simulink model "VFlexP_small"  (R2026a)
settings: Solver=ode23tb  StopTime=2  FixedStep=5e-5
model workspace (MAT data in the model file):
  DCop_DCBUCK : object (value not decoded)
  Grid_CCVSC_idx = [2; 3; 4; 5; 6; 7; 8; 9; 10; 11; 12]
  Grid_CCVSCs = 1
  Grid_CCVSCs_buses = 1
  Grid_CCVSCs_toM = [0 1 0 0 0 0 0 0 0 0 0 0 ... (781 elements, 71x11)]
  Grid_C_Lines = 0
  Grid_Cbuses = [0.00666666666667 0.00666666666667]
  Grid_DC : object (value not decoded)
  Grid_DCop_DCBUCK : object (value not decoded)
  Grid_DCop_DC_PES : object (value not decoded)
  Grid_DFIGs = 1
  Grid_DFIGs_buses = 1
  Grid_DGs : string (value not decoded)
  Grid_From_buses = 1
  Grid_GFls = 1
  Grid_GFls_buses = 1
  Grid_GFr_idx = 1
  Grid_GFrs = 1
  Grid_GFrs_buses = 1
  Grid_GFrs_toM = [1; 0]
  Grid_IG_idx = 1
  Grid_IGs = 1
  Grid_IGs_buses = 1
  Grid_IGs_toM = [1; 0; 0]
  Grid_L_Lines = 0.05
  Grid_L_Loads = [0 0]
  Grid_Lines_fromM : object (value not decoded)
  Grid_Lines_toM : object (value not decoded)
  Grid_Load_buses = [1; 2]
  Grid_Load_busesDC = []
  Grid_MSGs = 1
  Grid_MSGs_buses = 1
  Grid_Nbuses = 2
  Grid_PQ_gen = 3
  Grid_Ploads = [0.0075 0.0075]
  Grid_PloadsDC = []
  Grid_Ps_lf = 0.51232912
  Grid_Qloads = [0 0]
  Grid_Qs_lf = -0.00723209333333
  Grid_R_Lines = 0.005
  Grid_R_Loads = [2 2]
  Grid_R_Loads_DC = 0
  Grid_Rcf = [150 150]
  Grid_SCs = 1
  Grid_SCs_buses = 1
  Grid_SG_idx = 1
  Grid_SGs = 1
  Grid_SGs_buses = 1
  Grid_SGs_toM = [1; 0]
  Grid_To_buses = 2
  Grid_VCVSC_idx = [1; 2; 3; 4; 5; 6; 7; 8; 9; 10; 11; 12]
  Grid_VCVSCs = 1
  Grid_VCVSCs_buses = [1; 2; 3; 6; 8; 9; 12; 58; 59; 60; 63; 65]
  Grid_VCVSCs_toM = [1 0 0 0 0 0 0 0 0 0 0 0 ... (852 elements, 71x12)]
  Grid_VSM_idx = 2
  Grid_VSMs = 1
  Grid_VSMs_buses = 1
  Grid_VSMs_toM = [0; 1]
  Grid_admitt_matrix = [2.15353135314-19.7953135314i  -1.9801980198+19.801980198i; -1.9801980198+19.801980198i  2.15353135314-19.7953135314i]
  Grid_admitt_matrix_noloads = [1.98686468647-19.7953135314i  -1.9801980198+19.801980198i; -1.9801980198+19.801980198i  1.98686468647-19.7953135314i]
  Grid_bus = [1; 2]
  Grid_busDC_complexity = 1
  Grid_busDC_complexity_PF = 2
  Grid_bus_complexity = [1 1]
  Grid_bus_complexity_PF = [1 1]
  Grid_buses_lf = 1
  Grid_conductance_matrix = 0.00666666666667
  Grid_conductance_matrix_noloads = 0.00666666666667
  Grid_fref : object (value not decoded)
  Grid_gen_static_params : mBase (value not decoded)
  Grid_iPs_lf = 1.95187031336
  Grid_iQs_lf = -138.272551792
  Grid_iadmitt_matrix = [2.88165849328-0.0982918688642i  2.87905051706-0.123273862303i; 2.87905051706-0.123273862303i  2.88165849328-0.0982918688642i]
  Grid_iadmitt_matrix_noloads = [37.5012524798-37.4874983544i  37.4987475202-37.5125016456i; 37.4987475202-37.5125016456i  37.5012524798-37.4874983544i]
  Grid_iconductance_matrix = 150
  Grid_iconductance_matrix_noloads = 150
  Grid_init_OK_bool = 1
  Grid_intconv_PF : object (value not decoded)
  Grid_lf_op : op_report (value not decoded)
  Grid_lineDC_complexity = []
  Grid_lineDC_complexity_PF = []
  Grid_line_complexity = 1
  Grid_line_complexity_PF = 3
  Grid_loadDC_complexity = []
  Grid_loadDC_complexity_PF = []
  Grid_load_complexity = [3 3]
  Grid_load_complexity_PF = [4 4]
  Grid_opDC_CCVSC : object (value not decoded)
  Grid_opDC_VSM : object (value not decoded)
  Grid_opGFr : object (value not decoded)
  Grid_opVCVSC : object (value not decoded)
  Grid_op_CCVSC : object (value not decoded)
  Grid_op_IG : object (value not decoded)
  Grid_op_SG : object (value not decoded)
  Grid_op_VSM : object (value not decoded)
  Grid_shift_lines = 0
  Grid_tap_lines = 1
  Grid_v_buses_mod = [1 1]
  LinsysParamChangeStruct : Param1 (value not decoded)
  Lline = 0.01
  Rline = 1e-05
  linsys : object (value not decoded)
values from neighbouring files (symbols this model uses):
  block_idx = evalin(mdlWks, [bvarname Generators{i} '_idx'])    [fun_init_units_callback.m]
  Fb = areas    [fun_MATPOWER_to_Excel.m]
  Fi = evalin('base', get_param(block, 'Fi'))    [fun_init_GFr.m]    (also in fun_init_intconv_DC_VSM.m)
  Lf = evalin('base', get_param(block, 'Lf'))    [fun_init_GFr.m]    (also in fun_init_intconv_DC_VSM.m)
  Rf = evalin('base', get_param(block, 'Rf'))    [fun_init_GFr.m]    (also in fun_init_intconv_DC_VSM.m)
symbols that are objects in the model workspace (value not decoded): Grid_DCop_DC_PES, Grid_DCop_DCBUCK, Grid_op_CCVSC, Grid_op_IG, Grid_op_SG, Grid_op_VSM, Grid_opDC_CCVSC, Grid_opDC_VSM, Grid_opGFr, Grid_opVCVSC
undefined symbols (not defined in the file or in its folder): block_buses_DC, CCVSC_idx, Cf, costs, costs2, DFIGs_nodes, DiscIntNeverNeededParam, entity, From_nodes, grid_linsys, Grid_op_DFIG, Grid_op_DFIG_PQ, Grid_op_MSG, Grid_op_SC, Grid_op_VCVSC, Hv, initial_states_grid, Kic, Kiv, Kp_theta, Kp_w, Kpc, Kpv, last_send, Lc, m, Matrix_flux_to_i, mD, mp, MSGs_buses, Nbuses_DC, nq, op_VCVSC, Psche, Rc, rkq1, rkq2, SCs_buses, SCs_nodes, sec_control_structure, set_asked, set_DG_up, set_extra_satur, set_sending_cost, SGs_buses, SGs_nodes, Tf, To_nodes, VI_L, VI_R, WOF_Tf, xkq1, xkq2
libraries: simulink x1045, eeGeneralControl x12, eeTransforms x1, sl_discontinuities x1
(part 25 of 50)

== system VFlexP_small/Grid/Loadflow/Loads/dynamic/to_all_Loads1 ==
  In1 : Inport
  Assignment : Assignment  DiagnosticForDimensions=Warning  IndexOptions=Index vector (dialog)  Indices=find(load_complexity_PF == 1)  OutputSizes=1
  Zero : Constant  Value=zeros(1,length(L_Loads))  VectorParams1D=off  OutDataTypeStr=Inherit: Inherit via back propagation
  id : Outport
  wires:
  Assignment/1 -> id/1
  In1/1 -> Assignment/2
  Zero/1 -> Assignment/1

== system VFlexP_small/Grid/Loadflow/Loads/dynamic PQ/to_all_Loads ==
  In1 : Inport
  Assignment : Assignment  DiagnosticForDimensions=Warning  IndexOptions=Index vector (dialog)  Indices=find(load_complexity_PF == 5)  OutputSizes=1
  Zero : Constant  Value=zeros(1,length(L_Loads))  VectorParams1D=off  OutDataTypeStr=Inherit: Inherit via back propagation
  Out1 : Outport
  wires:
  Zero/1 -> Assignment/1
  In1/1 -> Assignment/2
  Assignment/1 -> Out1/1

== system VFlexP_small/Grid/Loadflow/Loads/dynamic PQ/to_all_Loads1 ==
  In1 : Inport
  Assignment : Assignment  DiagnosticForDimensions=Warning  IndexOptions=Index vector (dialog)  Indices=find(load_complexity_PF == 5)  OutputSizes=1
  Zero : Constant  Value=zeros(1,length(L_Loads))  VectorParams1D=off  OutDataTypeStr=Inherit: Inherit via back propagation
  Out1 : Outport
  wires:
  Assignment/1 -> Out1/1
  In1/1 -> Assignment/2
  Zero/1 -> Assignment/1

== system VFlexP_small/Grid/Loadflow/Loads/static/to_all_Loads ==
  In1 : Inport
  Assignment : Assignment  DiagnosticForDimensions=Warning  IndexOptions=Index vector (dialog)  Indices=find(load_complexity_PF == 2)  OutputSizes=1
  Zero : Constant  Value=zeros(1,length(L_Loads))  VectorParams1D=off  OutDataTypeStr=Inherit: Inherit via back propagation
  id : Outport
  wires:
  Zero/1 -> Assignment/1
  In1/1 -> Assignment/2
  Assignment/1 -> id/1

== system VFlexP_small/Grid/Loadflow/Loads/static/to_all_Loads1 ==
  In1 : Inport
  Assignment : Assignment  DiagnosticForDimensions=Warning  IndexOptions=Index vector (dialog)  Indices=find(load_complexity_PF == 2)  OutputSizes=1
  Zero : Constant  Value=zeros(1,length(L_Loads))  VectorParams1D=off  OutDataTypeStr=Inherit: Inherit via back propagation
  id : Outport
  wires:
  Assignment/1 -> id/1
  In1/1 -> Assignment/2
  Zero/1 -> Assignment/1

== system VFlexP_small/Grid/Loadflow/Loads/static omega/to_all_Loads ==
  In1 : Inport
  Assignment : Assignment  DiagnosticForDimensions=Warning  IndexOptions=Index vector (dialog)  Indices=find(load_complexity_PF == 3)  OutputSizes=1
  Zero : Constant  Value=zeros(1,length(L_Loads))  VectorParams1D=off  OutDataTypeStr=Inherit: Inherit via back propagation
  id : Outport
  wires:
  Zero/1 -> Assignment/1
  In1/1 -> Assignment/2
  Assignment/1 -> id/1

== system VFlexP_small/Grid/Loadflow/Loads/static omega/to_all_Loads1 ==
  In1 : Inport
  Assignment : Assignment  DiagnosticForDimensions=Warning  IndexOptions=Index vector (dialog)  Indices=find(load_complexity_PF == 3)  OutputSizes=1
  Zero : Constant  Value=zeros(1,length(L_Loads))  VectorParams1D=off  OutDataTypeStr=Inherit: Inherit via back propagation
  id : Outport
  wires:
  Assignment/1 -> id/1
  In1/1 -> Assignment/2
  Zero/1 -> Assignment/1

== system VFlexP_small/Grid/Dynamic/DCAC converters/DC_CCVSC/CC/dynamic ==
  idref : Inport
  iqref : Inport  Port=2
  vod : Inport  Port=3
  voq : Inport  Port=4
  omega : Inport  Port=5
  "Lf " : Gain  Gain=dparams.Lf
  Lf1 : Gain  Gain=dparams.Lf
  PId : Subsystem
  PIq : Subsystem
  Product : Product
  Product3 : Product
  RL : Subsystem  Variant=on  VariantControlMode=label  LabelModeActiveChoice=dynamic  mask(Line){dynamic=Dynamic, R=dparams.Rf, L=dparams.Lf, fbase=fb}
      mask prompts: dynamic "Dynamic behavior"; R "Series resistance (p.u.)"; L "Inductance (p.u.)"; fbase "Base frequency (Hz)"
      mask init: same as VFlexP_small/Grid/Loadflow/Generators/RL out
      mask Help: web('Documentation/RL.html')
      mask TypeOptions dynamic: Static | Dynamic | Static omega
  Sum1 : Sum  Inputs=++|
  Sum2 : Sum  Inputs=++|
  Sum8 : Sum  Inputs=-+|
  Sum9 : Sum  Inputs=|++
  idiref : Outport
  iqiref : Outport  Port=2
  vid : Outport  Port=3
  viq : Outport  Port=4
  wires:
  PId/1(Out1) -> Sum8/2
  idref/1 -> PId/1(ref)  "idref"
  RL/1(id) -> idiref/1, Lf1/1, PId/2(y)
  Sum2/1 -> viq/1, RL/3(v_in_q)
  Sum1/1 -> vid/1, RL/1(v_in_d)
  [voq] -> RL/4(v_out_q)
  [vod] -> RL/2(v_out_d)
  vod/1 -> [vod]  "iod"
  voq/1 -> [voq]  "ioq"
  omega/1 -> [omega]  "omega"
  [voq] -> Sum2/1
  [vod] -> Sum1/1
  Sum9/1 -> Sum2/2
  Sum8/1 -> Sum1/2
  iqref/1 -> PIq/1(ref)  "iqref"
  Product/1 -> Sum8/1
  [omega] -> Product/2
  Lf1/1 -> Product3/2
  Product3/1 -> Sum9/2
  "Lf "/1 -> Product/1
  [omega] -> Product3/1  "omega"
  PIq/1(Out1) -> Sum9/1
  RL/2(iq) -> "Lf "/1, PIq/2(y), iqiref/1
  [omega] -> RL/5(omega)  "omega"

== system VFlexP_small/Grid/Dynamic/DCAC converters/DC_CCVSC/CC/static ==
  idref : Inport
  iqref : Inport  Port=2
  vod : Inport  Port=3
  voq : Inport  Port=4
  omega : Inport  Port=5
  Terminator2 : Terminator
  idiref : Outport
  iqiref : Outport  Port=2
  vid : Outport  Port=3
  viq : Outport  Port=4
  wires:
  omega/1 -> Terminator2/1  "omega"
  iqref/1 -> iqiref/1  "iqref"
  idref/1 -> idiref/1  "idref"
  vod/1 -> vid/1  "vod"
  voq/1 -> viq/1  "voq"

== system VFlexP_small/Grid/Dynamic/DCAC converters/DC_CCVSC/PC/LPF_d ==
  In1 : Inport
  Gain : Gain  Gain=iTf
  I : Integrator  InitialCondition=v_buses_mod(block_buses)
  Sum4 : Sum  Inputs=|+-
  Out1 : Outport
  wires:
  I/1 -> Out1/1, Sum4/2
  In1/1 -> Sum4/1
  Sum4/1 -> Gain/1
  Gain/1 -> I/1

== system VFlexP_small/Grid/Dynamic/DCAC converters/DC_CCVSC/PC/LPF_q ==
  In1 : Inport
  Gain : Gain  Gain=iTf
  I : Integrator
  Sum4 : Sum  Inputs=|+-
  Out1 : Outport
  wires:
  Sum4/1 -> Gain/1
  In1/1 -> Sum4/1
  I/1 -> Out1/1, Sum4/2
  Gain/1 -> I/1

== system VFlexP_small/Grid/Dynamic/DCAC converters/DC_CCVSC/PC/Saturation ==
  ildref : Inport
  ilqref : Inport  Port=2
  Abs : Abs  ZeroCross=off  SaturateOnIntegerOverflow=off
  Abs1 : Abs  ZeroCross=off  SaturateOnIntegerOverflow=off
  Abs2 : Abs  ZeroCross=off  SaturateOnIntegerOverflow=off
  Divide2 : Product  Inputs=*/
  Divide3 : Product  Inputs=*/
  Gain : Gain  Gain=-1
  Gain3 : Gain  Gain=-1
  Real-Imag to Complex : RealImagToComplex
  Saturation Dynamic : simulink/Discontinuities/Saturation Dynamic  OutMin=[]  OutMax=[]  OutDataTypeStr=Inherit: Same as second input  OutDataType=fixdt(1, 16)  OutScaling=2^-10  DoSatur=off
  Saturation Dynamic1 : simulink/Discontinuities/Saturation Dynamic  OutMin=[]  OutMax=[]  OutDataTypeStr=Inherit: Same as second input  OutDataType=fixdt(1, 16)  OutScaling=2^-10  DoSatur=off
  y : Outport
  y1 : Outport  Port=2
  wires:
  Saturation Dynamic1/1 -> y1/1
  ildref/1 -> Real-Imag to Complex/1, Saturation Dynamic/2, Abs2/1
  Abs2/1 -> Divide2/1
  ilqref/1 -> Real-Imag to Complex/2, Saturation Dynamic1/2, Abs1/1
  Real-Imag to Complex/1 -> Abs/1
  Abs1/1 -> Divide3/1
  Gain3/1 -> Saturation Dynamic/3
  Abs/1 -> Divide2/2, Divide3/2
  Saturation Dynamic/1 -> y/1
  Divide2/1 -> Saturation Dynamic/1, Gain3/1
  Divide3/1 -> Saturation Dynamic1/1, Gain/1
  Gain/1 -> Saturation Dynamic1/3

== system VFlexP_small/Grid/Dynamic/DCAC converters/DC_CCVSC/PLL/dynamic ==
  vq : Inport
  omega : Inport  Port=2
  voutangle : Inport  Port=3
  PLL : Subsystem
  Product : Product
  Selector8 : Selector  InputPortWidth=length(fref.ref_units)  IndexOptions=Index vector (dialog)  Indices=block_fref  OutputSizes=1
  Sum2 : Sum  Inputs=|-+
  Sum3 : Sum  Inputs=+-|
  Terminator : Terminator
  Zero : Constant  Value=0  OutDataTypeStr=Inherit: Inherit via back propagation
  frame : Integrator  InitialCondition=Grid_opDC_CCVSC.frame  UpperSaturationLimit=pi  LowerSaturationLimit=-pi
  theta : Outport
  omega_point : Outport  Port=2
  wires:
  Sum2/1 -> PLL/1(In1)
  Sum3/1 -> Product/1
  PLL/1(Input2) -> Sum3/1, omega_point/1  "omega2"
  Product/1 -> frame/1
  frame/1 -> theta/1  "theta"
  Zero/1 -> Sum2/1
  omega/1 -> Sum3/2  "omega"
  vq/1 -> Sum2/2  "vq"
  voutangle/1 -> Terminator/1
  [omega_base] -> Selector8/1
  Selector8/1 -> Product/2

== system VFlexP_small/Grid/Dynamic/DCAC converters/DC_CCVSC/PLL/static ==
  vq : Inport
  omega : Inport  Port=2
  voutangle : Inport  Port=3
  Gain : Gain  Gain=-1
  Terminator : Terminator
  Terminator1 : Terminator
  Transport Delay : TransportDelay  DelayTime=1e-6  TransDelayFeedthrough=on
  theta : Outport
  omega_point : Outport  Port=2
  wires:
  voutangle/1 -> Gain/1
  omega/1 -> Terminator1/1, omega_point/1  "vq"
  vq/1 -> Terminator/1  "vq"
  Gain/1 -> Transport Delay/1
  Transport Delay/1 -> theta/1

== system VFlexP_small/Grid/Dynamic/DCAC converters/DC_VCVSC/PC/LPF_P ==
  P : Inport
  Gain : Gain  Gain=iTf
  I : Integrator  InitialCondition=Grid_op_VCVSC.States(5,:)
  Sum4 : Sum  Inputs=|+-
  P_f : Outport
  wires:
  I/1 -> Sum4/2, P_f/1
  P/1 -> Sum4/1
  Sum4/1 -> Gain/1
  Gain/1 -> I/1

== system VFlexP_small/Grid/Dynamic/DCAC converters/DC_VCVSC/PC/LPF_Q ==
  Q : Inport
  Gain : Gain  Gain=iTf
  I : Integrator  InitialCondition=Grid_op_VCVSC.States(6,:)
  Sum4 : Sum  Inputs=|+-
  Q_f : Outport
  wires:
  Sum4/1 -> Gain/1
  I/1 -> Sum4/2, Q_f/1
  Q/1 -> Sum4/1
  Gain/1 -> I/1

== system VFlexP_small/Grid/Dynamic/DCAC converters/DC_VCVSC/RL out/dynamic ==
  v_in_d : Inport
  v_out_d : Inport  Port=2
  v_in_q : Inport  Port=3
  v_out_q : Inport  Port=4
  Gain1 : Gain  Gain=L
  Gain2 : Gain  Gain=R
  Gain3 : Gain  Gain=R
  Gain4 : Gain  Gain=L
  Gain5 : Gain  Gain=invL*omegab
  Gain7 : Gain  Gain=invL*omegab
  Product : Product
  Product1 : Product
  Sum4 : Sum  Inputs=+-|
  Sum5 : Sum  Inputs=|-+
  Sum6 : Sum  Inputs=|++
  Sum7 : Sum  Inputs=-+|
  Sum8 : Sum  Inputs=|+-
  Sum9 : Sum  Inputs=-+|
  i_d : Integrator  InitialCondition=Grid_op_VCVSC.States(9,:)
  i_q : Integrator  InitialCondition=Grid_op_VCVSC.States(10,:)
  id : Outport
  iq : Outport  Port=2
  v_outd : Outport  Port=3
  v_outq : Outport  Port=4
  wires:
  v_in_q/1 -> Sum5/2  "v_in_q"
  v_in_d/1 -> Sum4/1  "v_in_d"
  Gain2/1 -> Sum4/2
  i_d/1 -> Gain2/1, Gain1/1, id/1  "id"
  Sum6/1 -> Gain5/1
  [omega_ref] -> Product1/1, Product/2  "omega"
  Gain5/1 -> i_d/1
  Product/1 -> Sum6/2
  Sum8/1 -> Gain7/1
  Sum4/1 -> Sum7/2
  Product1/1 -> Sum8/2
  Gain4/1 -> Product/1
  Sum7/1 -> Sum6/1
  Gain3/1 -> Sum5/1
  Sum5/1 -> Sum9/2
  Gain7/1 -> i_q/1
  i_q/1 -> Gain3/1, Gain4/1, iq/1  "iq"
  Gain1/1 -> Product1/2
  Sum9/1 -> Sum8/1
  v_out_d/1 -> Sum7/1, v_outd/1  "v_out_d"
  v_out_q/1 -> Sum9/1, v_outq/1  "v_out_q"

== system VFlexP_small/Grid/Dynamic/DCAC converters/DC_VCVSC/RL out/static ==
  v_in_d : Inport
  v_out_d : Inport  Port=2
  v_in_q : Inport  Port=3
  v_out_q : Inport  Port=4
  Constant : Constant  Value=R.^2
  Constant1 : Constant
  Divide : Product  Inputs=*/
  Gain : Gain  Gain=L
  Gain1 : Gain  Gain=R
  Gain2 : Gain  Gain=R
  Product{,1..5} (6 alike) : Product
  Sum : Sum  Inputs=|++
  Sum1 : Sum  Inputs=|+-
  Sum2 : Sum  Inputs=|+-
  Sum3 : Sum  Inputs=|++
  Sum4 : Sum  Inputs=|-+
  id : Outport
  iq : Outport  Port=2
  v_outd : Outport  Port=3
  v_outq : Outport  Port=4
  wires:
  v_in_q/1 -> Sum2/1  "v_in_q"
  v_out_d/1 -> Sum1/2, v_outd/1  "v_out_d"
  Sum/1 -> Divide/2
  Gain2/1 -> Product5/2
  Product/1 -> Sum/2
  Product1/1 -> Sum3/1
  Product5/1 -> Sum4/2
  Constant/1 -> Sum/1
  Sum2/1 -> Product3/2, Product5/1  "vq"
  Gain/1 -> Product2/2, Product/1, Product/2
  Constant1/1 -> Divide/1
  Product3/1 -> Sum3/2
  Sum1/1 -> Product4/1, Product1/1  "vd"
  Divide/1 -> Product2/1, Gain1/1, Gain2/1
  Product4/1 -> Sum4/1
  Product2/1 -> Product3/1, Product4/2
  Gain1/1 -> Product1/2
  Sum3/1 -> id/1  "id"
  Sum4/1 -> iq/1  "iq"
  v_out_q/1 -> Sum2/2, v_outq/1  "v_out_q"
  v_in_d/1 -> Sum1/1  "v_in_d"
  [omega_ref] -> Gain/1  "omega"

== system VFlexP_small/Grid/Dynamic/DCAC converters/DC_VCVSC/RL out/static_omega ==
  v_in_d : Inport
  v_out_d : Inport  Port=2
  v_in_q : Inport  Port=3
  v_out_q : Inport  Port=4
  Gain : Gain  Gain=1./(R.^2+L.^2)
  Gain2 : Gain  Gain=1./(R.^2+L.^2)
  Gain3 : Gain  Gain=R
  Gain4 : Gain  Gain=L
  Gain5 : Gain  Gain=L
  Gain6 : Gain  Gain=R
  Sum : Sum  Inputs=|++
  Sum1 : Sum  Inputs=|+-
  Sum2 : Sum  Inputs=|+-
  Sum3 : Sum  Inputs=|-+
  id : Outport
  iq : Outport  Port=2
  v_outd : Outport  Port=3
  v_outq : Outport  Port=4
  wires:
  Gain6/1 -> Sum3/2
  Sum3/1 -> iq/1
  Gain5/1 -> Sum3/1
  Sum/1 -> id/1
  Gain2/1 -> Gain4/1, Gain6/1
  Gain4/1 -> Sum/2
  Gain3/1 -> Sum/1
  Gain/1 -> Gain3/1, Gain5/1
  Sum2/1 -> Gain2/1  "vq"
  Sum1/1 -> Gain/1  "vd"
  v_out_d/1 -> Sum1/2, v_outd/1  "v_out_d"
  v_out_q/1 -> Sum2/2, v_outq/1  "v_out_q"
  v_in_d/1 -> Sum1/1  "v_in_d"
  v_in_q/1 -> Sum2/1  "v_in_q"

== system VFlexP_small/Grid/Dynamic/DCAC converters/DC_VCVSC/VCC/dynamic ==
  vodref : Inport
  voqref : Inport  Port=2
  iod : Inport  Port=3
  ioq : Inport  Port=4
  omega : Inport  Port=5
  Cf : Gain  Gain=Cfi
  Cf 1 : Gain  Gain=Cfi
  Fi : Gain  Gain=Fi
  Fi2 : Gain  Gain=Fi
  "Lf " : Gain  Gain=Lf
  Lf1 : Gain  Gain=Lf
  Product{,1..3} (4 alike) : Product
  RC : Subsystem  Variant=on  VariantControlMode=label  LabelModeActiveChoice=dynamic  mask{dynamic=Dynamic, R=Rcf, C=Cfi, fbase=50}
      mask prompts: dynamic "Dynamic behavior"; R "Parallel resistance (p.u.)"; C "Capacitance (p.u.)"; fbase "Base frequency (Hz)"
      mask init:
      | omegab = 2*pi*fbase;
      | iC = 1./C;
      | iR = 1./R;
      | vssBlk = gcb;
      | switch dynamic
      |     case "Dynamic"
      |         set_param(vssBlk, 'LabelModeActiveChoice', 'dynamic');
      |     case "Static"
      |         set_param(vssBlk, 'LabelModeActiveChoice', 'static');
      |     case "Static omega"
      |         set_param(vssBlk, 'LabelModeActiveChoice', 'static omega');
      | end
      mask TypeOptions dynamic: Dynamic | Static | Static omega
  RL : Subsystem  Variant=on  VariantControlMode=label  LabelModeActiveChoice=dynamic  mask(Line){dynamic=Dynamic, R=Rf, L=Lf, fbase=fb}
      mask prompts: dynamic "Dynamic behavior"; R "Series resistance (p.u.)"; L "Inductance (p.u.)"; fbase "Base frequency (Hz)"
      mask init: same as VFlexP_small/Grid/Loadflow/Generators/RL out
      mask Help: web('Documentation/RL.html')
      mask TypeOptions dynamic: Static | Dynamic | Static omega
  Subsystem : Subsystem
  Subsystem1 : Subsystem
  Subsystem2 : Subsystem
  Subsystem3 : Subsystem
  Sum1 : Sum  Inputs=++|
  Sum2 : Sum  Inputs=-+|
  Sum{3,5..6,9} (4 alike) : Sum  Inputs=|++
  Sum4 : Sum  Inputs=++|
  Sum8 : Sum  Inputs=-+|
  vidref : Outport
  viqref : Outport  Port=2
  wires:
  Sum6/1 -> RL/3(v_in_q)
  Sum1/1 -> RL/1(v_in_d)
  Sum9/1 -> Sum6/1  "viqref"
  Sum8/1 -> Sum1/2  "vidref"
  RL/2(iq) -> "Lf "/1, Subsystem3/2(y), RC/3(i_q_in)
  RL/1(id) -> RC/1(i_d_in), Lf1/1, Subsystem2/2(y)
  RC/1(v_d) -> Cf 1/1, Subsystem/2(y), RL/2(v_out_d), Sum1/1, vidref/1
  [omega] -> Product1/1
  omega/1 -> [omega], Product2/1  "omega"
  Subsystem3/1(Out1) -> Sum9/1
  Subsystem2/1(Out1) -> Sum8/2
  Subsystem1/1(Out1) -> Sum3/1
  Subsystem/1(Out1) -> Sum2/2
  Fi2/1 -> Sum5/2
  ioq/1 -> Fi2/1, RC/4(i_q_out)  "ioq"
  [omega] -> Product3/1, RC/5(omega)  "omega"
  Sum3/1 -> Sum5/1
  "Lf "/1 -> Product/1
  Sum2/1 -> Sum4/2
  iod/1 -> Fi/1, RC/2(i_d_out)  "iod"
  Product1/1 -> Sum2/1
  Sum4/1 -> Subsystem2/1(ref)  "ildref"
  Cf/1 -> Product1/2
  Cf 1/1 -> Product2/2
  Product2/1 -> Sum3/2
  Product3/1 -> Sum9/2
  voqref/1 -> Subsystem1/1(ref)  "voqref"
  Fi/1 -> Sum4/1
  Lf1/1 -> Product3/2
  [omega] -> Product/2
  RC/2(v_q) -> Cf/1, Subsystem1/2(y), RL/4(v_out_q), Sum6/2, viqref/1  "voq"
  vodref/1 -> Subsystem/1(ref)  "vodref"
  Product/1 -> Sum8/1
  Sum5/1 -> Subsystem3/1(ref)  "ilqref"

== system VFlexP_small/Grid/Dynamic/DCAC converters/DC_VCVSC/VCC/dynamic_VC ==
  vodref : Inport
  voqref : Inport  Port=2
  iod : Inport  Port=3
  ioq : Inport  Port=4
  omega : Inport  Port=5
  Cf : Gain  Gain=Cfi
  Cf 1 : Gain  Gain=Cfi
  Fi : Gain  Gain=Fi
  Fi2 : Gain  Gain=Fi
  Product1 : Product
  Product2 : Product
  RC : Subsystem  Variant=on  VariantControlMode=label  LabelModeActiveChoice=dynamic  mask{dynamic=Dynamic, R=Rcf, C=Cfi, fbase=50}
      mask prompts: dynamic "Dynamic behavior"; R "Parallel resistance (p.u.)"; C "Capacitance (p.u.)"; fbase "Base frequency (Hz)"
      mask init: same as VFlexP_small/Grid/Dynamic/DCAC converters/DC_VCVSC/VCC/dynamic/RC
      mask TypeOptions dynamic: Dynamic | Static | Static omega
  Subsystem : Subsystem
  Subsystem1 : Subsystem
  Sum2 : Sum  Inputs=-+|
  Sum3 : Sum  Inputs=|++
  Sum4 : Sum  Inputs=++|
  Sum5 : Sum  Inputs=|++
  vidref : Outport
  viqref : Outport  Port=2
  wires:
  Sum5/1 -> RC/3(i_q_in)
  Sum4/1 -> RC/1(i_d_in)
  RC/1(v_d) -> Subsystem/2(y), Cf 1/1, vidref/1
  vodref/1 -> Subsystem/1(ref)  "vodref"
  RC/2(v_q) -> Subsystem1/2(y), Cf/1, viqref/1
  Fi/1 -> Sum4/1
  voqref/1 -> Subsystem1/1(ref)  "voqref"
  Product2/1 -> Sum3/2
  Cf 1/1 -> Product2/2
  Cf/1 -> Product1/2
  Product1/1 -> Sum2/1
  iod/1 -> Fi/1, RC/2(i_d_out)  "iod"
  Sum2/1 -> Sum4/2
  Sum3/1 -> Sum5/1
  ioq/1 -> Fi2/1, RC/4(i_q_out)  "ioq"
  Fi2/1 -> Sum5/2
  Subsystem/1(Out1) -> Sum2/2
  Subsystem1/1(Out1) -> Sum3/1
  omega/1 -> [omega], Product2/1, RC/5(omega)  "omega"
  [omega] -> Product1/1

== system VFlexP_small/Grid/Dynamic/DCAC converters/DC_VCVSC/VCC/dynamic_limiting ==
  note: Current limiting, no priority
  vodref : Inport
  voqref : Inport  Port=2
  iod : Inport  Port=3
  ioq : Inport  Port=4
  omega : Inport  Port=5
  Abs : Abs  ZeroCross=off  SaturateOnIntegerOverflow=off
  Abs1 : Abs  ZeroCross=off  SaturateOnIntegerOverflow=off
  Abs2 : Abs  ZeroCross=off  SaturateOnIntegerOverflow=off
  Cf : Gain  Gain=Cfi
  Cf 1 : Gain  Gain=Cfi
  Divide : Product  Inputs=*/
  Divide1 : Product  Inputs=*/
  Fi : Gain  Gain=Fi
  Fi2 : Gain  Gain=Fi
  Gain : Gain  Gain=-1
  Gain1 : Gain  Gain=-1
  "Lf " : Gain  Gain=Lf
  Lf1 : Gain  Gain=Lf
  Memory : Memory  InitialCondition=1  LinearizeMemory=on
  Memory1 : Memory  InitialCondition=1  LinearizeMemory=on
  PIi_d : Subsystem
  PIi_q : Subsystem
  PIv_d : Subsystem
  PIv_q : Subsystem
  Product{,1..3} (4 alike) : Product
  RC : Subsystem  Variant=on  VariantControlMode=label  LabelModeActiveChoice=dynamic  mask{dynamic=Dynamic, R=Rcf, C=Cfi, fbase=50}
      mask prompts: dynamic "Dynamic behavior"; R "Parallel resistance (p.u.)"; C "Capacitance (p.u.)"; fbase "Base frequency (Hz)"
      mask init: same as VFlexP_small/Grid/Dynamic/DCAC converters/DC_VCVSC/VCC/dynamic/RC
      mask TypeOptions dynamic: Dynamic | Static | Static omega
  RL : Subsystem  Variant=on  VariantControlMode=label  LabelModeActiveChoice=dynamic  mask(Line){dynamic=Dynamic, R=Rf, L=Lf, fbase=fb}
      mask prompts: dynamic "Dynamic behavior"; R "Series resistance (p.u.)"; L "Inductance (p.u.)"; fbase "Base frequency (Hz)"
      mask init: same as VFlexP_small/Grid/Loadflow/Generators/RL out
      mask Help: web('Documentation/RL.html')
      mask TypeOptions dynamic: Static | Dynamic | Static omega
  Real-Imag to Complex : RealImagToComplex
  Relational Operator : RelationalOperator  Operator===  OutDataTypeStr=boolean  ZeroCross=off  RndMeth=Simplest  InputSameDT=off
  Relational Operator1 : RelationalOperator  Operator===  OutDataTypeStr=boolean  ZeroCross=off  RndMeth=Simplest  InputSameDT=off
  Saturation Dynamic : simulink/Discontinuities/Saturation Dynamic  OutMin=[]  OutMax=[]  OutDataTypeStr=Inherit: Same as second input  OutDataType=fixdt(1, 16)  OutScaling=2^-10  DoSatur=off
  Saturation Dynamic1 : simulink/Discontinuities/Saturation Dynamic  OutMin=[]  OutMax=[]  OutDataTypeStr=Inherit: Same as second input  OutDataType=fixdt(1, 16)  OutScaling=2^-10  DoSatur=off
  Sum : Sum  Inputs=|+-
  Sum{1..2,6,8} (4 alike) : Sum  Inputs=-+|
  Sum3 : Sum  Inputs=|++
  Sum4 : Sum  Inputs=++|
  Sum5 : Sum  Inputs=|++
  Sum7 : Sum  Inputs=|+-
  Sum9 : Sum  Inputs=|++
  vidref : Outport
  viqref : Outport  Port=2
  wires:
  Memory/1 -> PIv_d/2(In2)
  Memory1/1 -> PIv_q/2(In2)
  Relational Operator1/1 -> Memory1/1
  Sum/1 -> PIv_q/1(In1)
  Relational Operator/1 -> Memory/1
  Sum1/1 -> PIv_d/1(In1)
  Gain1/1 -> Saturation Dynamic/3
  Gain/1 -> Saturation Dynamic1/3
  Divide1/1 -> Saturation Dynamic1/1, Gain/1
  Divide/1 -> Saturation Dynamic/1, Gain1/1
  Abs/1 -> Divide/2, Divide1/2
  Real-Imag to Complex/1 -> Abs/1
  Sum5/1 -> Real-Imag to Complex/2, Saturation Dynamic1/2, Abs1/1, Relational Operator1/1  "ilqref"
  Product/1 -> Sum8/1
  vodref/1 -> Sum1/2  "vodref"
  RC/2(v_q) -> viqref/1, RL/4(v_out_q), Sum/2, Cf/1  "voq"
  [omega] -> Product/2
  Lf1/1 -> Product3/2
  Fi/1 -> Sum4/1
  Sum6/1 -> PIi_d/1(In1)
  voqref/1 -> Sum/1  "voqref"
  Product3/1 -> Sum9/2
  Product2/1 -> Sum3/2
  Cf 1/1 -> Product2/2
  Cf/1 -> Product1/2
  Sum4/1 -> Real-Imag to Complex/1, Saturation Dynamic/2, Abs2/1, Relational Operator/1  "ildref"
  Product1/1 -> Sum2/1
  iod/1 -> RC/2(i_d_out), Fi/1  "iod"
  Sum2/1 -> Sum4/2
  Sum7/1 -> PIi_q/1(In1)
  "Lf "/1 -> Product/1
  Sum3/1 -> Sum5/1
  [omega] -> RC/5(omega), Product3/1  "omega"
  ioq/1 -> RC/4(i_q_out), Fi2/1  "ioq"
  Fi2/1 -> Sum5/2
  PIv_d/1(Out1) -> Sum2/2
  PIv_q/1(Out1) -> Sum3/1
  PIi_d/1(Out1) -> Sum8/2
  PIi_q/1(Out1) -> Sum9/1
  omega/1 -> Product2/1, [omega]  "omega"
  [omega] -> Product1/1
  RC/1(v_d) -> vidref/1, RL/2(v_out_d), Cf 1/1, Sum1/1
  RL/1(id) -> Lf1/1, Sum6/1, RC/1(i_d_in)
  RL/2(iq) -> RC/3(i_q_in), "Lf "/1, Sum7/2
  Sum8/1 -> RL/1(v_in_d)  "vidref"
  Sum9/1 -> RL/3(v_in_q)  "viqref"
  Abs1/1 -> Divide1/1
  Abs2/1 -> Divide/1
  Saturation Dynamic1/1 -> Relational Operator1/2, Sum7/1
  Saturation Dynamic/1 -> Relational Operator/2, Sum6/2

== system VFlexP_small/Grid/Dynamic/DCAC converters/DC_VCVSC/VCC/static ==
  vodref : Inport
  voqref : Inport  Port=2
  iod : Inport  Port=3
  ioq : Inport  Port=4
  omega : Inport  Port=5
  Terminator : Terminator
  Terminator1 : Terminator
  Terminator2 : Terminator
  vidref : Outport
  viqref : Outport  Port=2
  wires:
  omega/1 -> Terminator2/1  "ioq"
  ioq/1 -> Terminator1/1  "ioq"
  iod/1 -> Terminator/1  "iod"
  vodref/1 -> vidref/1  "vodref"
  voqref/1 -> viqref/1  "voqref"

== system VFlexP_small/Grid/Dynamic/DCAC converters/DC_VCVSC/VI/WOF_d ==
  In1 : Inport
  Gain : Gain  Gain=iTf
  I : Integrator  InitialConditionSource=external  InitialCondition=Grid_op_VCVSC.op.States(6).x'
  Sum : Sum  Inputs=+-|
  Sum4 : Sum  Inputs=|+-
  Out1 : Outport
  wires:
  Gain/1 -> I/1
  Sum4/1 -> Gain/1
  In1/1 -> I/2, Sum/1, Sum4/1
  I/1 -> Sum/2, Sum4/2
  Sum/1 -> Out1/1

== system VFlexP_small/Grid/Dynamic/DCAC converters/DC_VCVSC/VI/WOF_q ==
  In1 : Inport
  Gain : Gain  Gain=iTf
  I : Integrator  InitialConditionSource=external  InitialCondition=Grid_op_VCVSC.op.States(7).x'
  Sum : Sum  Inputs=+-|
  Sum4 : Sum  Inputs=|+-
  Out1 : Outport
  wires:
  Gain/1 -> I/1
  Sum4/1 -> Gain/1
  In1/1 -> I/2, Sum/1, Sum4/1
  I/1 -> Sum/2, Sum4/2
  Sum/1 -> Out1/1

== system VFlexP_small/Grid/Dynamic/DCAC converters/DC_VSM/PC/LPF_P ==
  P : Inport
  Gain : Gain  Gain=1e4
  I : Integrator  InitialCondition=Grid_opDC_VSM.P
  Sum4 : Sum  Inputs=|+-
  P_f : Outport
  wires:
  Gain/1 -> I/1
  Sum4/1 -> Gain/1
  P/1 -> Sum4/1
  I/1 -> P_f/1, Sum4/2

== system VFlexP_small/Grid/Dynamic/DCAC converters/DC_VSM/PC/LPF_P2 ==
  P : Inport
  Gain : Gain  Gain=1e4
  I : Integrator  InitialCondition=Grid_opDC_VSM.P
  Sum4 : Sum  Inputs=|+-
  P_f : Outport
  wires:
  I/1 -> Sum4/2, P_f/1
  P/1 -> Sum4/1
  Sum4/1 -> Gain/1
  Gain/1 -> I/1

== system VFlexP_small/Grid/Dynamic/DCAC converters/DC_VSM/PC/LPF_Q ==
  Q : Inport
  Gain : Gain  Gain=iTf
  I : Integrator
  Sum4 : Sum  Inputs=|+-
  Q_f : Outport
  wires:
  Gain/1 -> I/1
  Q/1 -> Sum4/1
  I/1 -> Q_f/1, Sum4/2
  Sum4/1 -> Gain/1

== system VFlexP_small/Grid/Dynamic/DCAC converters/DC_VSM/PC/Turbine model ==
  In1 : Inport
  Out1 : Outport
  wires:
  In1/1 -> Out1/1

== system VFlexP_small/Grid/Dynamic/DCAC converters/DC_VSM/PC/WOF_d ==
  In1 : Inport
  Gain : Gain  Gain=10
  Gain1 : Gain  Gain=10
  I : Integrator  InitialConditionSource=external  InitialCondition=Grid_op_VSM.op.States(7).x'
  Sum : Sum  Inputs=+-|
  Sum4 : Sum  Inputs=|+-
  Out1 : Outport
  wires:
  Gain/1 -> I/1
  Sum4/1 -> Gain/1
  In1/1 -> I/2, Sum/1, Sum4/1
  I/1 -> Sum/2, Sum4/2
  Sum/1 -> Gain1/1
  Gain1/1 -> Out1/1

== system VFlexP_small/Grid/Dynamic/DCAC converters/DC_VSM/RL out/dynamic ==
  v_in_d : Inport
  v_out_d : Inport  Port=2
  v_in_q : Inport  Port=3
  v_out_q : Inport  Port=4
  Gain1 : Gain  Gain=L
  Gain2 : Gain  Gain=R
  Gain3 : Gain  Gain=R
  Gain4 : Gain  Gain=L
  Gain5 : Gain  Gain=invL*omegab
  Gain7 : Gain  Gain=invL*omegab
  Product : Product
  Product1 : Product
  Sum4 : Sum  Inputs=+-|
  Sum5 : Sum  Inputs=|-+
  Sum6 : Sum  Inputs=|++
  Sum7 : Sum  Inputs=-+|
  Sum8 : Sum  Inputs=|+-
  Sum9 : Sum  Inputs=-+|
  i_d : Integrator  InitialCondition=Grid_opDC_VSM.id_out
  i_q : Integrator  InitialCondition=Grid_opDC_VSM.iq_out
  id : Outport
  iq : Outport  Port=2
  v_outd : Outport  Port=3
  v_outq : Outport  Port=4
  wires:
  v_out_q/1 -> v_outq/1, Sum9/1  "v_out_q"
  v_out_d/1 -> v_outd/1, Sum7/1  "v_out_d"
  Sum9/1 -> Sum8/1
  Gain1/1 -> Product1/2
  i_q/1 -> iq/1, Gain4/1, Gain3/1  "iq"
  Gain7/1 -> i_q/1
  Sum5/1 -> Sum9/2
  Gain3/1 -> Sum5/1
  Sum7/1 -> Sum6/1
  Gain4/1 -> Product/1
  Product1/1 -> Sum8/2
  Sum4/1 -> Sum7/2
  Sum8/1 -> Gain7/1
  Product/1 -> Sum6/2
  Gain5/1 -> i_d/1
  [omega_ref] -> Product/2, Product1/1  "omega"
  Sum6/1 -> Gain5/1
  i_d/1 -> id/1, Gain1/1, Gain2/1  "id"
  Gain2/1 -> Sum4/2
  v_in_d/1 -> Sum4/1  "v_in_d"
  v_in_q/1 -> Sum5/2  "v_in_q"

== system VFlexP_small/Grid/Dynamic/DCAC converters/DC_VSM/RL out/static ==
  v_in_d : Inport
  v_out_d : Inport  Port=2
  v_in_q : Inport  Port=3
  v_out_q : Inport  Port=4
  Constant : Constant  Value=R.^2
  Constant1 : Constant
  Divide : Product  Inputs=*/
  Gain : Gain  Gain=L
  Gain1 : Gain  Gain=R
  Gain2 : Gain  Gain=R
  Product{,1..5} (6 alike) : Product
  Sum : Sum  Inputs=|++
  Sum1 : Sum  Inputs=|+-
  Sum2 : Sum  Inputs=|+-
  Sum3 : Sum  Inputs=|++
  Sum4 : Sum  Inputs=|-+
  id : Outport
  iq : Outport  Port=2
  v_outd : Outport  Port=3
  v_outq : Outport  Port=4
  wires:
  [omega_ref] -> Gain/1  "omega"
  v_in_d/1 -> Sum1/1  "v_in_d"
  v_out_q/1 -> v_outq/1, Sum2/2  "v_out_q"
  Sum4/1 -> iq/1  "iq"
  Sum3/1 -> id/1  "id"
  Gain1/1 -> Product1/2
  Product2/1 -> Product4/2, Product3/1
  Product4/1 -> Sum4/1
  Divide/1 -> Gain2/1, Gain1/1, Product2/1
  Sum1/1 -> Product1/1, Product4/1  "vd"
  Product3/1 -> Sum3/2
  Constant1/1 -> Divide/1
  Gain/1 -> Product/2, Product/1, Product2/2
  Sum2/1 -> Product5/1, Product3/2  "vq"
  Constant/1 -> Sum/1
  Product5/1 -> Sum4/2
  Product1/1 -> Sum3/1
  Product/1 -> Sum/2
  Gain2/1 -> Product5/2
  Sum/1 -> Divide/2
  v_out_d/1 -> v_outd/1, Sum1/2  "v_out_d"
  v_in_q/1 -> Sum2/1  "v_in_q"

== system VFlexP_small/Grid/Dynamic/DCAC converters/DC_VSM/RL out/static_omega ==
  v_in_d : Inport
  v_out_d : Inport  Port=2
  v_in_q : Inport  Port=3
  v_out_q : Inport  Port=4
  Gain : Gain  Gain=1./(R.^2+L.^2)
  Gain2 : Gain  Gain=1./(R.^2+L.^2)
  Gain3 : Gain  Gain=R
  Gain4 : Gain  Gain=L
  Gain5 : Gain  Gain=L
  Gain6 : Gain  Gain=R
  Sum : Sum  Inputs=|++
  Sum1 : Sum  Inputs=|+-
  Sum2 : Sum  Inputs=|+-
  Sum3 : Sum  Inputs=|-+
  id : Outport
  iq : Outport  Port=2
  v_outd : Outport  Port=3
  v_outq : Outport  Port=4
  wires:
  v_in_q/1 -> Sum2/1  "v_in_q"
  v_in_d/1 -> Sum1/1  "v_in_d"
  v_out_q/1 -> v_outq/1, Sum2/2  "v_out_q"
  v_out_d/1 -> v_outd/1, Sum1/2  "v_out_d"
  Sum1/1 -> Gain/1  "vd"
  Sum2/1 -> Gain2/1  "vq"
  Gain/1 -> Gain5/1, Gain3/1
  Gain3/1 -> Sum/1
  Gain4/1 -> Sum/2
  Gain2/1 -> Gain6/1, Gain4/1
  Sum/1 -> id/1
  Gain5/1 -> Sum3/1
  Sum3/1 -> iq/1
  Gain6/1 -> Sum3/2

== system VFlexP_small/Grid/Dynamic/DCAC converters/DC_VSM/VCC/dynamic ==
  vodref : Inport
  voqref : Inport  Port=2
  iod : Inport  Port=3
  ioq : Inport  Port=4
  omega : Inport  Port=5
  Cf : Gain  Gain=Cfi
  Cf 1 : Gain  Gain=Cfi
  Fi : Gain  Gain=Fi
  Fi2 : Gain  Gain=Fi
  "Lf " : Gain  Gain=Lf
  Lf1 : Gain  Gain=Lf
  PIid : Subsystem
  PIiq : Subsystem
  PIvd : Subsystem
  PIvq : Subsystem
  Product{,1..3} (4 alike) : Product
  RC : Subsystem  Variant=on  VariantControlMode=label  LabelModeActiveChoice=dynamic  mask{dynamic=Dynamic, R=Rcf, C=Cfi, fbase=50}
      mask prompts: dynamic "Dynamic behavior"; R "Parallel resistance (p.u.)"; C "Capacitance (p.u.)"; fbase "Base frequency (Hz)"
      mask init: same as VFlexP_small/Grid/Dynamic/DCAC converters/DC_VCVSC/VCC/dynamic/RC
      mask TypeOptions dynamic: Dynamic | Static | Static omega
  RL : Subsystem  Variant=on  VariantControlMode=label  LabelModeActiveChoice=dynamic  mask(Line){dynamic=Dynamic, R=Rf, L=Lf, fbase=fb}
      mask prompts: dynamic "Dynamic behavior"; R "Series resistance (p.u.)"; L "Inductance (p.u.)"; fbase "Base frequency (Hz)"
      mask init: same as VFlexP_small/Grid/Loadflow/Generators/RL out
      mask Help: web('Documentation/RL.html')
      mask TypeOptions dynamic: Static | Dynamic | Static omega
  Sum1 : Sum  Inputs=++|
  Sum2 : Sum  Inputs=-+|
  Sum{3,5..6,9} (4 alike) : Sum  Inputs=|++
  Sum4 : Sum  Inputs=++|
  Sum8 : Sum  Inputs=-+|
  vidref : Outport
  viqref : Outport  Port=2
  wires:
  Sum5/1 -> PIiq/1(ref)  "ilqref"
  Product/1 -> Sum8/1
  vodref/1 -> PIvd/1(ref)  "vodref"
  RC/2(vq) -> viqref/1, Sum6/2, RL/4(v_out_q), PIvq/2(y), Cf/1  "voq"
  [omega] -> Product/2
  Lf1/1 -> Product3/2
  Fi/1 -> Sum4/1
  voqref/1 -> PIvq/1(ref)  "voqref"
  Product3/1 -> Sum9/2
  Product2/1 -> Sum3/2
  Cf 1/1 -> Product2/2
  Cf/1 -> Product1/2
  Sum4/1 -> PIid/1(ref)  "ildref"
  Product1/1 -> Sum2/1
  iod/1 -> RC/2(i_d_out), Fi/1  "iod"
  Sum2/1 -> Sum4/2
  "Lf "/1 -> Product/1
  Sum3/1 -> Sum5/1
  [omega] -> RC/5(omega), Product3/1  "omega"
  ioq/1 -> RC/4(i_q_out), Fi2/1  "ioq"
  Fi2/1 -> Sum5/2
  PIvd/1(Out1) -> Sum2/2
  PIvq/1(Out1) -> Sum3/1
  PIid/1(Out1) -> Sum8/2
  PIiq/1(Out1) -> Sum9/1
  omega/1 -> Product2/1, [omega]  "omega"
  [omega] -> Product1/1
  RC/1(vd) -> vidref/1, Sum1/1, RL/2(v_out_d), PIvd/2(y), Cf 1/1
  RL/1(id) -> PIid/2(y), Lf1/1, RC/1(i_d_in)
  RL/2(iq) -> RC/3(i_q_in), PIiq/2(y), "Lf "/1
  Sum8/1 -> Sum1/2  "vidref"
  Sum9/1 -> Sum6/1  "viqref"
  Sum1/1 -> RL/1(v_in_d)
  Sum6/1 -> RL/3(v_in_q)

== system VFlexP_small/Grid/Dynamic/DCAC converters/DC_VSM/VCC/dynamic_VC ==
  vodref : Inport
  voqref : Inport  Port=2
  iod : Inport  Port=3
  ioq : Inport  Port=4
  omega : Inport  Port=5
  Cf : Gain  Gain=Cfi
  Cf 1 : Gain  Gain=Cfi
  Fi : Gain  Gain=Fi
  Fi2 : Gain  Gain=Fi
  Product1 : Product
  Product2 : Product
  RC : Subsystem  Variant=on  VariantControlMode=label  LabelModeActiveChoice=dynamic  mask{dynamic=Dynamic, R=Rcf, C=Cfi, fbase=50}
      mask prompts: dynamic "Dynamic behavior"; R "Parallel resistance (p.u.)"; C "Capacitance (p.u.)"; fbase "Base frequency (Hz)"
      mask init: same as VFlexP_small/Grid/Dynamic/DCAC converters/DC_VCVSC/VCC/dynamic/RC
      mask TypeOptions dynamic: Dynamic | Static | Static omega
  Subsystem : Subsystem
  Subsystem1 : Subsystem
  Sum2 : Sum  Inputs=-+|
  Sum3 : Sum  Inputs=|++
  Sum4 : Sum  Inputs=++|
  Sum5 : Sum  Inputs=|++
  vidref : Outport
  viqref : Outport  Port=2
  wires:
  [omega] -> Product1/1
  omega/1 -> RC/5(omega), Product2/1, [omega]  "omega"
  Subsystem1/1(Out1) -> Sum3/1
  Subsystem/1(Out1) -> Sum2/2
  Fi2/1 -> Sum5/2
  ioq/1 -> RC/4(i_q_out), Fi2/1  "ioq"
  Sum3/1 -> Sum5/1
  Sum2/1 -> Sum4/2
  iod/1 -> RC/2(i_d_out), Fi/1  "iod"
  Product1/1 -> Sum2/1
  Cf/1 -> Product1/2
  Cf 1/1 -> Product2/2
  Product2/1 -> Sum3/2
  voqref/1 -> Subsystem1/1(ref)  "voqref"
  Fi/1 -> Sum4/1
  RC/2(v_q) -> viqref/1, Cf/1, Subsystem1/2(y)
  vodref/1 -> Subsystem/1(ref)  "vodref"
  RC/1(v_d) -> vidref/1, Cf 1/1, Subsystem/2(y)
  Sum4/1 -> RC/1(i_d_in)
  Sum5/1 -> RC/3(i_q_in)

== system VFlexP_small/Grid/Dynamic/DCAC converters/DC_VSM/VCC/dynamic_limiting ==
  vodref : Inport
  voqref : Inport  Port=2
  iod : Inport  Port=3
  ioq : Inport  Port=4
  omega : Inport  Port=5
  Cf : Gain  Gain=Cfi
  Cf 1 : Gain  Gain=Cfi
  Complex to Magnitude-Angle2 : ComplexToMagnitudeAngle  Output=Magnitude
  Complex to Magnitude-Angle3 : ComplexToMagnitudeAngle
  Complex to Magnitude-Angle4 : ComplexToMagnitudeAngle  Output=Magnitude
  Complex to Magnitude-Angle5 : ComplexToMagnitudeAngle  Output=Magnitude
  Complex to Real-Imag1 : ComplexToRealImag
  Fi : Gain  Gain=Fi
  Fi2 : Gain  Gain=Fi
  "Lf " : Gain  Gain=Lf
  Lf1 : Gain  Gain=Lf
  Magnitude-Angle to Complex : MagnitudeAngleToComplex
  Memory : Memory
  NOT : Logic  Operator=NOT  IconShape=distinctive  AllPortsSameDT=off  OutDataTypeStr=boolean
  PIid : Subsystem
  PIiq : Subsystem
  PIvd : Subsystem
      settings: PortSchema="{\"entries\":[{\"content\":{\"sides\":[{\"content\":{\"connectorIds\":[\"In1\",\"In2\"]},\"type\":\"ConnectorPlacement.EquallySpacedRectSide\",\"uuid\":\"218efe14-094c-4cdd-8e62-ef6089c75bbd\"},{\"content\":{\"connectorIds\":[\"Out1\"],\"side\":\"RIGHT\"},\"type\":\"ConnectorPlacement.EquallySpacedRectSide\",\"uuid\":\"287e2a8a-062a-4519-a86c-f141c6982dac\"},{\"content\":{\"connectorIds\":[\"In3\"],\"side\":\"TOP\"},\"type\":\"ConnectorPlacement.EquallySpacedRectSide\",\"uuid\":\"e88fce21-908c-492a-b265-04b05ce94be8\"}]},\"type\":\"ConnectorPlacement.EquallySpacedConnector\",\"uuid\":\"5c149457-da6d-4223-b1cb-56365173b759\"}],\"packageUris\":[\"http://schema.mathworks.com/mf0/Connector/R2020b\"],\"version\":\"1.0\"}"
  PIvq : Subsystem
      settings: PortSchema="{\"entries\":[{\"content\":{\"sides\":[{\"content\":{\"connectorIds\":[\"In1\",\"In2\"]},\"type\":\"ConnectorPlacement.EquallySpacedRectSide\",\"uuid\":\"218efe14-094c-4cdd-8e62-ef6089c75bbd\"},{\"content\":{\"connectorIds\":[\"Out1\"],\"side\":\"RIGHT\"},\"type\":\"ConnectorPlacement.EquallySpacedRectSide\",\"uuid\":\"287e2a8a-062a-4519-a86c-f141c6982dac\"},{\"content\":{\"connectorIds\":[],\"side\":\"TOP\"},\"type\":\"ConnectorPlacement.EquallySpacedRectSide\",\"uuid\":\"e88fce21-908c-492a-b265-04b05ce94be8\"},{\"content\":{\"connectorIds\":[\"In3\"],\"side\":\"BOTTOM\"},\"type\":\"ConnectorPlacement.EquallySpacedRectSide\",\"uuid\":\"db964aea-37c6-4226-90b6-d177a6d2ab38\"}]},\"type\":\"ConnectorPlacement.EquallySpacedConnector\",\"uuid\":\"5c149457-da6d-4223-b1cb-56365173b759\"}],\"packageUris\":[\"http://schema.mathworks.com/mf0/Connector/R2020b\"],\"version\":\"1.0\"}"
  Product{,1..5} (6 alike) : Product
  RC : Subsystem  Variant=on  VariantControlMode=label  LabelModeActiveChoice=dynamic  mask{dynamic=Dynamic, R=Rcf, C=Cfi}
      mask prompts: dynamic "Dynamic behavior"; R "Parallel resistance (p.u.)"; C "Capacitance (p.u.)"
      mask init:
      | iC = 1./C;
      | iR = 1./R;
      | vssBlk = gcb;
      | switch dynamic
      |     case "Dynamic"
      |         set_param(vssBlk, 'LabelModeActiveChoice', 'dynamic');
      |     case "Static"
      |         set_param(vssBlk, 'LabelModeActiveChoice', 'static');
      |     case "Static omega"
      |         set_param(vssBlk, 'LabelModeActiveChoice', 'static omega');
      | end
      mask TypeOptions dynamic: Dynamic | Static | Static omega
  RL : Subsystem  Variant=on  VariantControlMode=label  LabelModeActiveChoice=dynamic  mask(Line){dynamic=Dynamic, R=Rf, L=Lf}
      mask prompts: dynamic "Dynamic behavior"; R "Series resistance (p.u.)"; L "Inductance (p.u.)"
      mask init: same as VFlexP_small/Grid/Dynamic/Generators/GFr/RL out
      mask Help: web('Documentation/RL.html')
      mask TypeOptions dynamic: Static | Dynamic | Static omega
  Real-Imag to Complex{2..5} (4 alike) : RealImagToComplex
  Relational Operator : RelationalOperator  Operator===  OutDataTypeStr=boolean  RndMeth=Simplest  InputSameDT=off
  Saturation : Saturate  UpperLimit=0.1  LowerLimit=0
  Scope{1,3,6..8} (5 alike) : Scope
      Scope1 settings: ActiveDisplayYMinimum=-0.06728  ActiveDisplayYMaximum=0.79818  DataLoggingVariableName=ScopeData2
      Scope3 settings: ActiveDisplayYMinimum=0.01769  ActiveDisplayYMaximum=0.10915
      Scope6 settings: ActiveDisplayYMinimum=0.03196  ActiveDisplayYMaximum=0.13112  DataLoggingVariableName=ScopeData2
      Scope7 settings: ActiveDisplayYMinimum=0.86043  ActiveDisplayYMaximum=1.1554  DataLoggingVariableName=ScopeData3
      Scope8 settings: ActiveDisplayYMinimum=0.0318  ActiveDisplayYMaximum=0.12782  DataLoggingVariableName=ScopeData4
  Scope2 : Scope  NumInputPorts=2
      settings: ActiveDisplayYMinimum=-0.10019  ActiveDisplayYMaximum=0.20176
  Scope4 : Scope  NumInputPorts=2
      settings: ActiveDisplayYMinimum=-0.04364  ActiveDisplayYMaximum=0.0791  DataLoggingVariableName=ScopeData3
  Sum1 : Sum  Inputs=++|
  Sum{3,5..6,9,14..15} (6 alike) : Sum  Inputs=|++
  Sum2 : Sum  Inputs=-+|
  Sum4 : Sum  Inputs=++|
  Sum8 : Sum  Inputs=-+|
  VI : Subsystem  mask{L=0.5, R=0.1, Tf=0}
      mask prompts: L "Inductance (pu)"; R "Resistance (pu)"; Tf "WOF time constant (s)"
      mask init: same as VFlexP_small/Grid/Dynamic/DCAC converters/DC_VCVSC/VI
  vidref : Outport
  viqref : Outport  Port=2
  wires:
  Product/1 -> Sum8/1
  Sum14/1 -> PIvd/1(ref)  "vodref"
  RC/2(vq) -> [voq], viqref/1, RL/4(v_out_q), Sum6/2, PIvq/2(y), Cf/1, Real-Imag to Complex4/2  "voq"
  [omega] -> Product/2
  Lf1/1 -> Product3/2
  Fi/1 -> Sum4/1
  Sum15/1 -> PIvq/1(ref)  "voqref"
  Product3/1 -> Sum9/2
  Product2/1 -> Sum3/2
  Cf 1/1 -> Product2/2
  Cf/1 -> Product1/2
  Product1/1 -> Sum2/1
  iod/1 -> RC/2(i_d_out), Real-Imag to Complex5/1, Product4/2, Fi/1  "iod"
  Sum2/1 -> Sum4/2
  "Lf "/1 -> Product/1
  Sum3/1 -> Sum5/1
  [omega] -> RC/5(omega), RL/5(omega), Product3/1  "omega"
  ioq/1 -> RC/4(i_q_out), Fi2/1, Real-Imag to Complex5/2, Product5/2  "ioq"
  Fi2/1 -> Sum5/2
  PIvd/1(Out1) -> Sum2/2
  PIvq/1(Out1) -> Sum3/1
  PIid/1(Out1) -> Sum8/2
  PIiq/1(Out1) -> Sum9/1
  omega/1 -> Product2/1, [omega]  "omega"
  [omega] -> Product1/1
  RL/1(id) -> RC/1(i_d_in), Scope2/1, Real-Imag to Complex2/1, PIid/2(y), Lf1/1
  RL/2(iq) -> Scope4/1, PIiq/2(y), "Lf "/1, Real-Imag to Complex2/2, RC/3(i_q_in)
  Sum8/1 -> Sum1/2  "vidref"
  Sum9/1 -> Sum6/1  "viqref"
  Sum1/1 -> RL/1(v_in_d)
  Sum6/1 -> RL/3(v_in_q)
  Sum4/1 -> Real-Imag to Complex3/1, [ildref]  "ildref"
  Sum5/1 -> Real-Imag to Complex3/2, [ilqref]  "ilqref"
  RC/1(vd) -> Real-Imag to Complex4/1, RL/2(v_out_d), Sum1/1, [vod], vidref/1, PIvd/2(y), Cf 1/1
  Complex to Real-Imag1/2 -> Scope4/2, PIiq/1(ref)
  Real-Imag to Complex2/1 -> Complex to Magnitude-Angle2/1
  Complex to Magnitude-Angle2/1 -> Scope1/1  "i_mod"
  Complex to Real-Imag1/1 -> Scope2/2, PIid/1(ref)
  Real-Imag to Complex3/1 -> Complex to Magnitude-Angle3/1
  Saturation/1 -> Magnitude-Angle to Complex/1, Scope3/1, Relational Operator/1
  Relational Operator/1 -> PIvd/3(anti_windup), PIvq/3(anti_windup), NOT/1
  Complex to Magnitude-Angle3/1 -> Scope6/1, Relational Operator/2, Saturation/1
  Magnitude-Angle to Complex/1 -> Complex to Real-Imag1/1
  Complex to Magnitude-Angle3/2 -> Magnitude-Angle to Complex/2
  Complex to Magnitude-Angle4/1 -> Scope7/1  "vc_mod"
  Real-Imag to Complex4/1 -> Complex to Magnitude-Angle4/1
  Real-Imag to Complex5/1 -> Complex to Magnitude-Angle5/1
  Complex to Magnitude-Angle5/1 -> Scope8/1  "io_mod"
  vodref/1 -> Sum14/2  "vodref"
  voqref/1 -> Sum15/1  "voqref"
  NOT/1 -> Memory/1
  VI/1(vd) -> Sum14/1
  VI/2(vq) -> Sum15/2
  Memory/1 -> Product5/1, Product4/1
  Product4/1 -> VI/1(id)
  Product5/1 -> VI/2(iq)
